simulink model "control_pos_6dof_conMI"  (R2023b)
settings: Solver=ode45  StartTime=0.0  StopTime=tsim  FixedStep=tstep  MaxStep=tstep
undefined symbols (not defined in the file): a0, a1, MI_Contr1, MI_Contr2, MI_Contr3, MI_Contr4, MI_Contr5, MI_Contr6, MI_motor1, MI_motor2, MI_motor3, MI_motor4, MI_motor5, MI_motor6, robot_params, sigbuilder_block, t_qeq_init, t_tr_init, tau_L, tr_ref
(part 1 of 10)
settings Model: Creator=HP  LastModifiedBy=HP

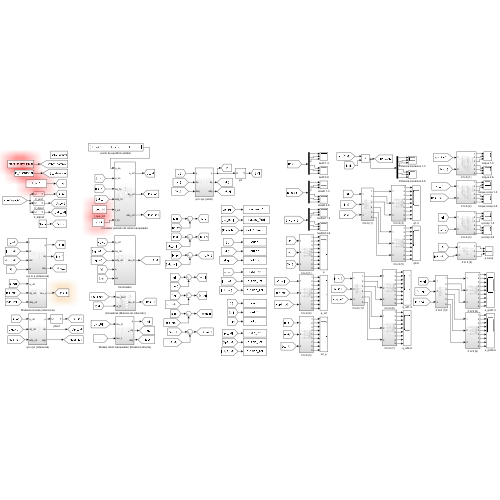
[thumbnail: Simulink's stored preview of the top-level diagram]
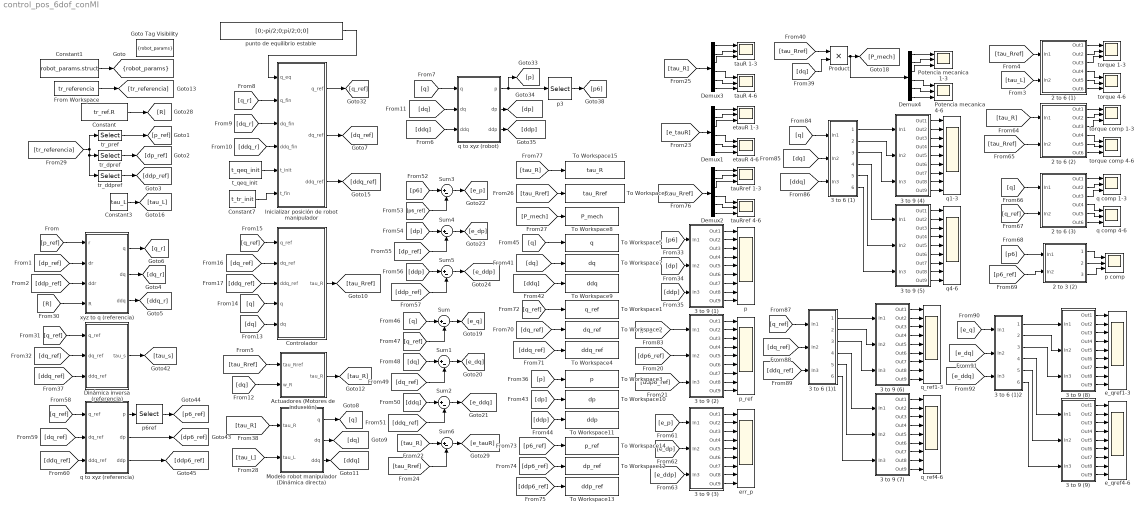
== system control_pos_6dof_conMI ==
  2 to 3 (2) : Subsystem
  2 to 6 (1) : Subsystem
  2 to 6 (2) : Subsystem
  2 to 6 (3) : Subsystem
  3 to 6 (1) : Subsystem
  3 to 6 (1)1 : Subsystem
  3 to 6 (1)2 : Subsystem
  3 to 9 (1) : Subsystem
  3 to 9 (2) : Subsystem
  3 to 9 (3) : Subsystem
  3 to 9 (4) : Subsystem
  3 to 9 (5) : Subsystem
  3 to 9 (6) : Subsystem
  3 to 9 (7) : Subsystem
  3 to 9 (8) : Subsystem
  3 to 9 (9) : Subsystem
  Actuadores (Motores de inducción) : Subsystem
  Constant : Constant  Value=tr_ref.R
  Constant1 : Constant  Value=robot_params.struct  OutDataTypeStr=Bus: robot_params_bus
  Constant3 : Constant  Value=tau_L
  Constant7 : Constant  Value=t_tr_init
  Controlador : Subsystem
  Demux{1..4} (4 alike) : Demux  Outputs=6
  Dinámica inversa (referencia) : Subsystem
  From Workspace : FromWorkspace  VariableName=tr_referencia
  Goto Tag Visibility : GotoTagVisibility  GotoTag=robot_params
  Inicializar posición de robot manipulador : Subsystem
  Modelo robot manipulador (Dinámica directa) : Subsystem
  Potencia mecanica 1-3 : Scope  NumInputPorts=3
  Potencia mecanica 4-6 : Scope  NumInputPorts=3
  Product : Product
  Sum{,1..6} (7 alike) : Sum  Inputs=|+-
  To Workspace1 : ToWorkspace  VariableName=q_ref  SaveFormat=Timeseries  SampleTime=-1
  To Workspace10 : ToWorkspace  VariableName=dp  SaveFormat=Timeseries  SampleTime=-1
  To Workspace11 : ToWorkspace  VariableName=ddp  SaveFormat=Timeseries  SampleTime=-1
  To Workspace12 : ToWorkspace  VariableName=dp_ref  SaveFormat=Timeseries  SampleTime=-1
  To Workspace13 : ToWorkspace  VariableName=ddp_ref  SaveFormat=Timeseries  SampleTime=-1
  To Workspace14 : ToWorkspace  VariableName=p_ref  SaveFormat=Timeseries  SampleTime=-1
  To Workspace15 : ToWorkspace  VariableName=tau_R  SaveFormat=Timeseries  SampleTime=-1
  To Workspace2 : ToWorkspace  VariableName=dq_ref  SaveFormat=Timeseries  SampleTime=-1
  To Workspace3 : ToWorkspace  VariableName=p  SaveFormat=Timeseries  SampleTime=-1
  To Workspace4 : ToWorkspace  VariableName=ddq_ref  SaveFormat=Timeseries  SampleTime=-1
  To Workspace5 : ToWorkspace  VariableName=q  SaveFormat=Timeseries  SampleTime=-1
  To Workspace6 : ToWorkspace  VariableName=tau_Rref  SaveFormat=Timeseries  SampleTime=-1
  To Workspace7 : ToWorkspace  VariableName=dq  SaveFormat=Timeseries  SampleTime=-1
  To Workspace8 : ToWorkspace  VariableName=P_mech  SaveFormat=Timeseries  SampleTime=-1
  To Workspace9 : ToWorkspace  VariableName=ddq  SaveFormat=Timeseries  SampleTime=-1
  e_qref1-3 : Scope  NumInputPorts=9
  e_qref4-6 : Scope  NumInputPorts=9
  err_p : Scope  NumInputPorts=9
  etauR 1-3 : Scope  NumInputPorts=3
  etauR 4-6 : Scope  NumInputPorts=3
  p : Scope  NumInputPorts=9
  p comp : Scope  NumInputPorts=3
  p3 : Selector  NumberOfDimensions=2  InputPortWidth=3  IndexOptions=Index vector (dialog),Index vector (dialog)  Indices=[1:3],6  OutputSizes=1,1
  p6ref : Selector  NumberOfDimensions=2  InputPortWidth=3  IndexOptions=Index vector (dialog),Index vector (dialog)  Indices=[1:3],6  OutputSizes=1,1
  p_ref : Scope  NumInputPorts=9
  punto de equilibrio estable : Constant  Value=[0;-pi/2;0;pi/2;0;0]
  q comp 1-3 : Scope  NumInputPorts=3
  q comp 4-6 : Scope  NumInputPorts=3
  q to xyz (referencia) : Subsystem
  q to xyz (robot) : Subsystem
  q1-3 : Scope  NumInputPorts=9
  q4-6 : Scope  NumInputPorts=9
  q_ref1-3 : Scope  NumInputPorts=9
  q_ref4-6 : Scope  NumInputPorts=9
  t_qeq_init : Constant  Value=t_qeq_init
  tauR 1-3 : Scope  NumInputPorts=3
  tauR 4-6 : Scope  NumInputPorts=3
  tauRref 1-3 : Scope  NumInputPorts=3
  tauRref 4-6 : Scope  NumInputPorts=3
  torque 1-3 : Scope  NumInputPorts=3
  torque 4-6 : Scope  NumInputPorts=3
  torque comp 1-3 : Scope  NumInputPorts=3
  torque comp 4-6 : Scope  NumInputPorts=3
  tr_ddpref : Selector  NumberOfDimensions=2  InputPortWidth=3  IndexOptions=Index vector (dialog),Index vector (dialog)  Indices=[7:9],1  OutputSizes=1,1
  tr_dpref : Selector  NumberOfDimensions=2  InputPortWidth=3  IndexOptions=Index vector (dialog),Index vector (dialog)  Indices=[4:6],1  OutputSizes=1,1
  tr_pref : Selector  NumberOfDimensions=2  InputPortWidth=3  IndexOptions=Index vector (dialog),Index vector (dialog)  Indices=[1:3],1  OutputSizes=1,1
  xyz to q (referencia) : Subsystem
  tag scope: robot_params=scoped
  wires:
  [tr_referencia] -> tr_dpref/1, tr_ddpref/1, tr_pref/1
  3 to 9 (1)/8(Out8) -> p/8
  [ddp] -> 3 to 9 (1)/3(In3)
  [dp] -> 3 to 9 (1)/2(In2)
  3 to 9 (1)/2(Out2) -> p/2
  [p6] -> 3 to 9 (1)/1(In1)
  3 to 9 (1)/7(Out7) -> p/7
  3 to 9 (1)/3(Out3) -> p/3
  3 to 9 (1)/5(Out5) -> p/5
  3 to 9 (1)/6(Out6) -> p/6
  3 to 9 (1)/9(Out9) -> p/9
  3 to 9 (1)/1(Out1) -> p/1
  3 to 9 (1)/4(Out4) -> p/4
  Constant3/1 -> [tau_L]
  [tau_Rref] -> Product/1
  [dq] -> Product/2
  [ddp] -> To Workspace11/1
  [P_mech] -> To Workspace8/1
  [dq] -> To Workspace7/1
  [q] -> To Workspace5/1
  [tau_Rref] -> To Workspace6/1
  [dp] -> To Workspace10/1
  [p] -> To Workspace3/1
  [ddq] -> To Workspace9/1
  [q] -> Sum/1
  [q_ref] -> Sum/2
  Sum/1 -> [e_q]
  [dq_ref] -> Sum1/2
  Sum1/1 -> [e_dq]
  [dq] -> Sum1/1
  [ddq_ref] -> Sum2/2
  Sum2/1 -> [e_ddq]
  [ddq] -> Sum2/1
  [p6_ref] -> Sum3/2
  Sum4/1 -> [e_dp]
  Sum5/1 -> [e_ddp]
  [ddp_ref] -> Sum5/2
  [dp_ref] -> Sum4/2
  Sum3/1 -> [e_p]
  [p6] -> Sum3/1
  [ddp] -> Sum5/1
  [dp] -> Sum4/1
  3 to 9 (3)/4(Out4) -> err_p/4
  3 to 9 (3)/1(Out1) -> err_p/1
  3 to 9 (3)/3(Out3) -> err_p/3
  3 to 9 (3)/7(Out7) -> err_p/7
  3 to 9 (3)/2(Out2) -> err_p/2
  3 to 9 (3)/6(Out6) -> err_p/6
  3 to 9 (3)/5(Out5) -> err_p/5
  [e_p] -> 3 to 9 (3)/1(In1)
  [e_dp] -> 3 to 9 (3)/2(In2)
  3 to 9 (3)/8(Out8) -> err_p/8
  3 to 9 (3)/9(Out9) -> err_p/9
  [e_ddp] -> 3 to 9 (3)/3(In3)
  [tau_R] -> 2 to 6 (2)/1(In1)
  [tau_Rref] -> 2 to 6 (2)/2(In2)
  [q_ref] -> 2 to 6 (3)/2(In2)
  [q] -> 2 to 6 (3)/1(In1)
  [p6] -> 2 to 3 (2)/1(In1)
  [p6_ref] -> 2 to 3 (2)/2(In2)
  [dq_ref] -> To Workspace2/1
  [ddq_ref] -> To Workspace4/1
  [q_ref] -> To Workspace1/1
  [p6_ref] -> To Workspace14/1
  [dp6_ref] -> To Workspace12/1
  [ddp6_ref] -> To Workspace13/1
  3 to 9 (2)/4(Out4) -> p_ref/4
  3 to 9 (2)/1(Out1) -> p_ref/1
  3 to 9 (2)/3(Out3) -> p_ref/3
  3 to 9 (2)/7(Out7) -> p_ref/7
  3 to 9 (2)/2(Out2) -> p_ref/2
  3 to 9 (2)/6(Out6) -> p_ref/6
  3 to 9 (2)/5(Out5) -> p_ref/5
  [p6_ref] -> 3 to 9 (2)/1(In1)
  3 to 9 (2)/8(Out8) -> p_ref/8
  3 to 9 (2)/9(Out9) -> p_ref/9
  2 to 6 (1)/3(Out3) -> torque 1-3/3
  2 to 6 (1)/2(Out2) -> torque 1-3/2
  2 to 6 (1)/1(Out1) -> torque 1-3/1
  [tau_R] -> Modelo robot manipulador (Dinámica directa)/1(tau_R)
  2 to 6 (1)/6(Out6) -> torque 4-6/3
  [tau_L] -> Modelo robot manipulador (Dinámica directa)/2(tau_L)
  2 to 6 (1)/5(Out5) -> torque 4-6/2
  2 to 6 (1)/4(Out4) -> torque 4-6/1
  Demux2/5 -> tauRref 4-6/2
  Demux2/4 -> tauRref 4-6/1
  [tau_Rref] -> Demux2/1
  Demux2/1 -> tauRref 1-3/1
  Demux2/2 -> tauRref 1-3/2
  Demux2/3 -> tauRref 1-3/3
  Demux2/6 -> tauRref 4-6/3
  3 to 9 (4)/5(Out5) -> q1-3/5
  3 to 9 (4)/2(Out2) -> q1-3/2
  3 to 6 (1)/1(Out1) -> 3 to 9 (4)/1(In1)
  3 to 9 (5)/5(Out5) -> q4-6/5
  3 to 9 (4)/3(Out3) -> q1-3/3
  3 to 9 (5)/3(Out3) -> q4-6/3
  3 to 9 (4)/4(Out4) -> q1-3/4
  3 to 9 (4)/8(Out8) -> q1-3/8
  3 to 9 (4)/7(Out7) -> q1-3/7
  3 to 9 (4)/6(Out6) -> q1-3/6
  3 to 9 (4)/9(Out9) -> q1-3/9
  3 to 9 (5)/1(Out1) -> q4-6/1
  3 to 9 (5)/6(Out6) -> q4-6/6
  3 to 9 (5)/7(Out7) -> q4-6/7
  3 to 9 (5)/4(Out4) -> q4-6/4
  3 to 9 (4)/1(Out1) -> q1-3/1
  3 to 9 (5)/8(Out8) -> q4-6/8
  [q] -> 3 to 6 (1)/1(In1)
  [dq] -> 3 to 6 (1)/2(In2)
  3 to 6 (1)/2(Out2) -> 3 to 9 (4)/2(In2)
  [ddq] -> 3 to 6 (1)/3(In3)
  3 to 6 (1)/3(Out3) -> 3 to 9 (4)/3(In3)
  3 to 9 (5)/2(Out2) -> q4-6/2
  3 to 6 (1)/6(Out6) -> 3 to 9 (5)/3(In3)
  3 to 6 (1)/5(Out5) -> 3 to 9 (5)/2(In2)
  3 to 6 (1)/4(Out4) -> 3 to 9 (5)/1(In1)
  [ddq_ref] -> 3 to 6 (1)1/3(In3)
  3 to 6 (1)1/3(Out3) -> 3 to 9 (6)/3(In3)
  [dq_ref] -> 3 to 6 (1)1/2(In2)
  [q_ref] -> 3 to 6 (1)1/1(In1)
  3 to 9 (7)/8(Out8) -> q_ref4-6/8
  3 to 9 (6)/1(Out1) -> q_ref1-3/1
  3 to 9 (7)/4(Out4) -> q_ref4-6/4
  3 to 6 (1)1/2(Out2) -> 3 to 9 (6)/2(In2)
  3 to 6 (1)1/5(Out5) -> 3 to 9 (7)/2(In2)
  3 to 9 (7)/2(Out2) -> q_ref4-6/2
  3 to 6 (1)1/6(Out6) -> 3 to 9 (7)/3(In3)
  3 to 9 (7)/7(Out7) -> q_ref4-6/7
  3 to 9 (7)/6(Out6) -> q_ref4-6/6
  3 to 9 (7)/1(Out1) -> q_ref4-6/1
  3 to 9 (6)/8(Out8) -> q_ref1-3/8
  3 to 9 (6)/6(Out6) -> q_ref1-3/6
  3 to 9 (6)/7(Out7) -> q_ref1-3/7
  3 to 9 (7)/5(Out5) -> q_ref4-6/5
  3 to 9 (6)/3(Out3) -> q_ref1-3/3
  3 to 9 (7)/3(Out3) -> q_ref4-6/3
  3 to 6 (1)1/1(Out1) -> 3 to 9 (6)/1(In1)
  3 to 9 (6)/2(Out2) -> q_ref1-3/2
  3 to 9 (6)/5(Out5) -> q_ref1-3/5
  3 to 9 (6)/9(Out9) -> q_ref1-3/9
  3 to 9 (6)/4(Out4) -> q_ref1-3/4
  3 to 6 (1)1/4(Out4) -> 3 to 9 (7)/1(In1)
  [e_ddq] -> 3 to 6 (1)2/3(In3)
  3 to 6 (1)2/3(Out3) -> 3 to 9 (8)/3(In3)
  [e_dq] -> 3 to 6 (1)2/2(In2)
  [e_q] -> 3 to 6 (1)2/1(In1)
  3 to 9 (9)/8(Out8) -> e_qref4-6/8
  3 to 9 (8)/1(Out1) -> e_qref1-3/1
  3 to 9 (9)/4(Out4) -> e_qref4-6/4
  3 to 6 (1)2/2(Out2) -> 3 to 9 (8)/2(In2)
  3 to 6 (1)2/5(Out5) -> 3 to 9 (9)/2(In2)
  3 to 9 (9)/2(Out2) -> e_qref4-6/2
  3 to 6 (1)2/6(Out6) -> 3 to 9 (9)/3(In3)
  3 to 9 (9)/7(Out7) -> e_qref4-6/7
  3 to 9 (9)/6(Out6) -> e_qref4-6/6
  3 to 9 (9)/1(Out1) -> e_qref4-6/1
  3 to 9 (8)/8(Out8) -> e_qref1-3/8
  3 to 9 (8)/6(Out6) -> e_qref1-3/6
  3 to 9 (8)/7(Out7) -> e_qref1-3/7
  3 to 9 (9)/5(Out5) -> e_qref4-6/5
  3 to 9 (8)/3(Out3) -> e_qref1-3/3
  3 to 9 (9)/3(Out3) -> e_qref4-6/3
  3 to 6 (1)2/1(Out1) -> 3 to 9 (8)/1(In1)
  3 to 9 (8)/2(Out2) -> e_qref1-3/2
  3 to 9 (8)/5(Out5) -> e_qref1-3/5
  3 to 9 (8)/9(Out9) -> e_qref1-3/9
  3 to 9 (8)/4(Out4) -> e_qref1-3/4
  3 to 6 (1)2/4(Out4) -> 3 to 9 (9)/1(In1)
  3 to 9 (5)/9(Out9) -> q4-6/9
  3 to 9 (7)/9(Out9) -> q_ref4-6/9
  3 to 9 (9)/9(Out9) -> e_qref4-6/9
  2 to 6 (2)/1(Out1) -> torque comp 1-3/1
  2 to 6 (2)/6(Out6) -> torque comp 4-6/3
  2 to 6 (2)/4(Out4) -> torque comp 4-6/1
  2 to 6 (2)/2(Out2) -> torque comp 1-3/2
  2 to 6 (2)/5(Out5) -> torque comp 4-6/2
  2 to 6 (2)/3(Out3) -> torque comp 1-3/3
  2 to 6 (3)/4(Out4) -> q comp 4-6/1
  2 to 6 (3)/2(Out2) -> q comp 1-3/2
  2 to 6 (3)/5(Out5) -> q comp 4-6/2
  2 to 6 (3)/3(Out3) -> q comp 1-3/3
  2 to 6 (3)/6(Out6) -> q comp 4-6/3
  2 to 6 (3)/1(Out1) -> q comp 1-3/1
  2 to 3 (2)/2(2) -> p comp/2
  2 to 3 (2)/1(1) -> p comp/1
  2 to 3 (2)/3(3) -> p comp/3
  Constant/1 -> [R]
  tr_pref/1 -> [p_ref]
  tr_ddpref/1 -> [ddp_ref]
  tr_dpref/1 -> [dp_ref]
  Constant1/1 -> [robot_params]
  [p_ref] -> xyz to q (referencia)/1(r)
  [dp_ref] -> xyz to q (referencia)/2(dr)
  [ddp_ref] -> xyz to q (referencia)/3(ddr)
  [R] -> xyz to q (referencia)/4(R)
  From Workspace/1 -> [tr_referencia]
  p3/1 -> [p6]
  q to xyz (robot)/1(p) -> p3/1, [p]
  [q] -> q to xyz (robot)/1(q)
  [dq] -> q to xyz (robot)/2(dq)
  [ddq] -> q to xyz (robot)/3(ddq)
  q to xyz (robot)/2(dp) -> [dp]
  q to xyz (robot)/3(ddp) -> [ddp]
  Modelo robot manipulador (Dinámica directa)/3(ddq) -> [ddq]
  Modelo robot manipulador (Dinámica directa)/2(dq) -> [dq]
  Modelo robot manipulador (Dinámica directa)/1(q) -> [q]
  [q_ref] -> Controlador/1(q_ref)
  [dq_ref] -> Controlador/2(dq_ref)
  [ddq_ref] -> Controlador/3(ddq_ref)
  [q] -> Controlador/4(q)
  [dq] -> Controlador/5(dq)
  Controlador/1(tau_R) -> [tau_Rref]
  [tau_Rref] -> 2 to 6 (1)/1(In1)
  [tau_L] -> 2 to 6 (1)/2(In2)
  xyz to q (referencia)/2(dq) -> [dq_r]
  xyz to q (referencia)/1(q) -> [q_r]
  xyz to q (referencia)/3(ddq) -> [ddq_r]
  [tau_Rref] -> Sum6/2
  [tau_R] -> Sum6/1
  Sum6/1 -> [e_tauR]
  [dp6_ref] -> 3 to 9 (2)/2(In2)
  [ddp6_ref] -> 3 to 9 (2)/3(In3)
  Demux1/1 -> etauR 1-3/1
  Demux1/3 -> etauR 1-3/3
  Demux1/6 -> etauR 4-6/3
  Demux1/2 -> etauR 1-3/2
  [e_tauR] -> Demux1/1
  Demux1/5 -> etauR 4-6/2
  Demux1/4 -> etauR 4-6/1
  Demux3/3 -> tauR 1-3/3
  Demux3/1 -> tauR 1-3/1
  Demux3/5 -> tauR 4-6/2
  Demux3/2 -> tauR 1-3/2
  Demux3/4 -> tauR 4-6/1
  Demux3/6 -> tauR 4-6/3
  [tau_R] -> Demux3/1
  Dinámica inversa (referencia)/1(tau_s) -> [tau_s]
  q to xyz (referencia)/2(dp) -> [dp6_ref]
  q to xyz (referencia)/3(ddp) -> [ddp6_ref]
  q to xyz (referencia)/1(p) -> p6ref/1
  p6ref/1 -> [p6_ref]
  [q_ref] -> Dinámica inversa (referencia)/1(q_ref)
  [dq_ref] -> Dinámica inversa (referencia)/2(dq_ref)
  [ddq_ref] -> Dinámica inversa (referencia)/3(ddq_ref)
  [q_ref] -> q to xyz (referencia)/1(q_ref)
  [dq_ref] -> q to xyz (referencia)/2(dq_ref)
  [ddq_ref] -> q to xyz (referencia)/3(ddq_ref)
  [tau_R] -> To Workspace15/1
  Demux4/6 -> Potencia mecanica 4-6/3
  Demux4/4 -> Potencia mecanica 4-6/1
  Product/1 -> Demux4/1, [P_mech]
  Demux4/3 -> Potencia mecanica 1-3/3
  Demux4/2 -> Potencia mecanica 1-3/2
  Demux4/1 -> Potencia mecanica 1-3/1
  Demux4/5 -> Potencia mecanica 4-6/2
  Constant7/1 -> Inicializar posición de robot manipulador/6(t_fin)
  [q_r] -> Inicializar posición de robot manipulador/2(q_fin)
  punto de equilibrio estable/1 -> Inicializar posición de robot manipulador/1(q_eq)
  Inicializar posición de robot manipulador/2(dq_ref) -> [dq_ref]
  t_qeq_init/1 -> Inicializar posición de robot manipulador/5(t_init)
  [ddq_r] -> Inicializar posición de robot manipulador/4(ddq_fin)
  Inicializar posición de robot manipulador/1(q_ref) -> [q_ref]
  Inicializar posición de robot manipulador/3(ddq_ref) -> [ddq_ref]
  [dq_r] -> Inicializar posición de robot manipulador/3(dq_fin)
  [tau_Rref] -> Actuadores (Motores de inducción)/1(tau_Rref)
  [dq] -> Actuadores (Motores de inducción)/2(w_R)
  Actuadores (Motores de inducción)/1(tau_R) -> [tau_R]

== system control_pos_6dof_conMI/2 to 3 (2) ==
  In1 : Inport
  In2 : Inport  Port=2
  Demux3 : Demux  Outputs=3
  Demux4 : Demux  Outputs=3
  Mux10 : Mux  Inputs=2
  Mux8 : Mux  Inputs=2
  Mux9 : Mux  Inputs=2
  1 : Outport
  2 : Outport  Port=2
  3 : Outport  Port=3
  wires:
  Demux4/3 -> Mux10/2
  Demux3/1 -> Mux8/1
  Demux3/2 -> Mux9/1
  Mux9/1 -> 2/1
  Demux4/2 -> Mux9/2
  Demux4/1 -> Mux8/2
  Demux3/3 -> Mux10/1
  Mux8/1 -> 1/1
  Mux10/1 -> 3/1
  In1/1 -> Demux3/1
  In2/1 -> Demux4/1

== system control_pos_6dof_conMI/2 to 6 (1) ==
  In1 : Inport
  In2 : Inport  Port=2
  Demux4 : Demux  Outputs=6
  Demux6 : Demux  Outputs=6
  Mux{,1..5} (6 alike) : Mux  Inputs=2
  Out1 : Outport
  Out2 : Outport  Port=2
  Out3 : Outport  Port=3
  Out4 : Outport  Port=4
  Out5 : Outport  Port=5
  Out6 : Outport  Port=6
  wires:
  In2/1 -> Demux6/1
  Demux4/3 -> Mux2/1
  Demux4/5 -> Mux4/1
  Demux4/6 -> Mux5/1
  Demux6/5 -> Mux4/2
  Demux4/1 -> Mux/1
  Demux6/6 -> Mux5/2
  In1/1 -> Demux4/1
  Demux4/4 -> Mux3/1
  Demux6/2 -> Mux1/2
  Demux6/4 -> Mux3/2
  Demux6/1 -> Mux/2
  Demux4/2 -> Mux1/1
  Demux6/3 -> Mux2/2
  Mux/1 -> Out1/1
  Mux1/1 -> Out2/1
  Mux2/1 -> Out3/1
  Mux3/1 -> Out4/1
  Mux4/1 -> Out5/1
  Mux5/1 -> Out6/1

== system control_pos_6dof_conMI/2 to 6 (2) ==
  In1 : Inport
  In2 : Inport  Port=2
  Demux4 : Demux  Outputs=6
  Demux6 : Demux  Outputs=6
  Mux{,1..5} (6 alike) : Mux  Inputs=2
  Out1 : Outport
  Out2 : Outport  Port=2
  Out3 : Outport  Port=3
  Out4 : Outport  Port=4
  Out5 : Outport  Port=5
  Out6 : Outport  Port=6
  wires:
  In2/1 -> Demux6/1
  Demux4/3 -> Mux2/1
  Demux4/5 -> Mux4/1
  Demux4/6 -> Mux5/1
  Demux6/5 -> Mux4/2
  Demux4/1 -> Mux/1
  Demux6/6 -> Mux5/2
  In1/1 -> Demux4/1
  Demux4/4 -> Mux3/1
  Demux6/2 -> Mux1/2
  Demux6/4 -> Mux3/2
  Demux6/1 -> Mux/2
  Demux4/2 -> Mux1/1
  Demux6/3 -> Mux2/2
  Mux/1 -> Out1/1
  Mux1/1 -> Out2/1
  Mux2/1 -> Out3/1
  Mux3/1 -> Out4/1
  Mux4/1 -> Out5/1
  Mux5/1 -> Out6/1

== system control_pos_6dof_conMI/2 to 6 (3) ==
  In1 : Inport
  In2 : Inport  Port=2
  Demux4 : Demux  Outputs=6
  Demux6 : Demux  Outputs=6
  Mux{,1..5} (6 alike) : Mux  Inputs=2
  Out1 : Outport
  Out2 : Outport  Port=2
  Out3 : Outport  Port=3
  Out4 : Outport  Port=4
  Out5 : Outport  Port=5
  Out6 : Outport  Port=6
  wires:
  In2/1 -> Demux6/1
  Demux4/3 -> Mux2/1
  Demux4/5 -> Mux4/1
  Demux4/6 -> Mux5/1
  Demux6/5 -> Mux4/2
  Demux4/1 -> Mux/1
  Demux6/6 -> Mux5/2
  In1/1 -> Demux4/1
  Demux4/4 -> Mux3/1
  Demux6/2 -> Mux1/2
  Demux6/4 -> Mux3/2
  Demux6/1 -> Mux/2
  Demux4/2 -> Mux1/1
  Demux6/3 -> Mux2/2
  Mux/1 -> Out1/1
  Mux1/1 -> Out2/1
  Mux2/1 -> Out3/1
  Mux3/1 -> Out4/1
  Mux4/1 -> Out5/1
  Mux5/1 -> Out6/1

== system control_pos_6dof_conMI/3 to 6 (1) ==
  In1 : Inport
  In2 : Inport  Port=2
  In3 : Inport  Port=3
  Demux4 : Demux  Outputs=6
  Demux6 : Demux  Outputs=6
  Demux7 : Demux  Outputs=6
  Mux{,1..5} (6 alike) : Mux  Inputs=3
  Out1 : Outport
  Out2 : Outport  Port=2
  Out3 : Outport  Port=3
  Out4 : Outport  Port=4
  Out5 : Outport  Port=5
  Out6 : Outport  Port=6
  wires:
  Demux6/1 -> Mux2/1
  Demux6/3 -> Mux2/3
  Demux4/2 -> Mux/2
  Demux6/6 -> Mux3/3
  Demux6/2 -> Mux2/2
  Demux6/5 -> Mux3/2
  Mux/1 -> Out1/1
  In1/1 -> Demux4/1
  Demux6/4 -> Mux3/1
  Demux4/1 -> Mux/1
  Demux4/6 -> Mux1/3
  Demux4/4 -> Mux1/1
  Demux7/5 -> Mux5/2
  Demux4/3 -> Mux/3
  Demux4/5 -> Mux1/2
  Demux7/3 -> Mux4/3
  Demux7/1 -> Mux4/1
  Demux7/2 -> Mux4/2
  In3/1 -> Demux7/1
  Mux2/1 -> Out2/1
  Demux7/4 -> Mux5/1
  Demux7/6 -> Mux5/3
  In2/1 -> Demux6/1
  Mux5/1 -> Out6/1
  Mux1/1 -> Out4/1
  Mux4/1 -> Out3/1
  Mux3/1 -> Out5/1

== system control_pos_6dof_conMI/3 to 6 (1)1 ==
  In1 : Inport
  In2 : Inport  Port=2
  In3 : Inport  Port=3
  Demux4 : Demux  Outputs=6
  Demux6 : Demux  Outputs=6
  Demux7 : Demux  Outputs=6
  Mux{,1..5} (6 alike) : Mux  Inputs=3
  Out1 : Outport
  Out2 : Outport  Port=2
  Out3 : Outport  Port=3
  Out4 : Outport  Port=4
  Out5 : Outport  Port=5
  Out6 : Outport  Port=6
  wires:
  Demux6/1 -> Mux2/1
  Demux6/3 -> Mux2/3
  Demux4/2 -> Mux/2
  Demux6/6 -> Mux3/3
  Demux6/2 -> Mux2/2
  Demux6/5 -> Mux3/2
  Mux/1 -> Out1/1
  In1/1 -> Demux4/1
  Demux6/4 -> Mux3/1
  Demux4/1 -> Mux/1
  Demux4/6 -> Mux1/3
  Demux4/4 -> Mux1/1
  Demux7/5 -> Mux5/2
  Demux4/3 -> Mux/3
  Demux4/5 -> Mux1/2
  Demux7/3 -> Mux4/3
  Demux7/1 -> Mux4/1
  Demux7/2 -> Mux4/2
  In3/1 -> Demux7/1
  Mux2/1 -> Out2/1
  Demux7/4 -> Mux5/1
  Demux7/6 -> Mux5/3
  In2/1 -> Demux6/1
  Mux5/1 -> Out6/1
  Mux1/1 -> Out4/1
  Mux4/1 -> Out3/1
  Mux3/1 -> Out5/1

== system control_pos_6dof_conMI/3 to 6 (1)2 ==
  In1 : Inport
  In2 : Inport  Port=2
  In3 : Inport  Port=3
  Demux4 : Demux  Outputs=6
  Demux6 : Demux  Outputs=6
  Demux7 : Demux  Outputs=6
  Mux{,1..5} (6 alike) : Mux  Inputs=3
  Out1 : Outport
  Out2 : Outport  Port=2
  Out3 : Outport  Port=3
  Out4 : Outport  Port=4
  Out5 : Outport  Port=5
  Out6 : Outport  Port=6
  wires:
  Demux6/1 -> Mux2/1
  Demux6/3 -> Mux2/3
  Demux4/2 -> Mux/2
  Demux6/6 -> Mux3/3
  Demux6/2 -> Mux2/2
  Demux6/5 -> Mux3/2
  Mux/1 -> Out1/1
  In1/1 -> Demux4/1
  Demux6/4 -> Mux3/1
  Demux4/1 -> Mux/1
  Demux4/6 -> Mux1/3
  Demux4/4 -> Mux1/1
  Demux7/5 -> Mux5/2
  Demux4/3 -> Mux/3
  Demux4/5 -> Mux1/2
  Demux7/3 -> Mux4/3
  Demux7/1 -> Mux4/1
  Demux7/2 -> Mux4/2
  In3/1 -> Demux7/1
  Mux2/1 -> Out2/1
  Demux7/4 -> Mux5/1
  Demux7/6 -> Mux5/3
  In2/1 -> Demux6/1
  Mux5/1 -> Out6/1
  Mux1/1 -> Out4/1
  Mux4/1 -> Out3/1
  Mux3/1 -> Out5/1

== system control_pos_6dof_conMI/3 to 9 (1) ==
  In1 : Inport
  In2 : Inport  Port=2
  In3 : Inport  Port=3
  Demux2 : Demux  Outputs=3
  Demux3 : Demux  Outputs=3
  Demux4 : Demux  Outputs=3
  Out1 : Outport
  Out2 : Outport  Port=2
  Out3 : Outport  Port=3
  Out4 : Outport  Port=4
  Out5 : Outport  Port=5
  Out6 : Outport  Port=6
  Out7 : Outport  Port=7
  Out8 : Outport  Port=8
  Out9 : Outport  Port=9
  wires:
  In3/1 -> Demux4/1
  Demux4/1 -> Out3/1
  Demux2/1 -> Out1/1
  Demux3/3 -> Out8/1
  Demux3/2 -> Out5/1
  Demux3/1 -> Out2/1
  In1/1 -> Demux2/1
  Demux2/3 -> Out7/1
  Demux4/3 -> Out9/1
  Demux4/2 -> Out6/1
  Demux2/2 -> Out4/1
  In2/1 -> Demux3/1

== system control_pos_6dof_conMI/3 to 9 (2) ==
  In1 : Inport
  In2 : Inport  Port=2
  In3 : Inport  Port=3
  Demux2 : Demux  Outputs=3
  Demux3 : Demux  Outputs=3
  Demux4 : Demux  Outputs=3
  Out1 : Outport
  Out2 : Outport  Port=2
  Out3 : Outport  Port=3
  Out4 : Outport  Port=4
  Out5 : Outport  Port=5
  Out6 : Outport  Port=6
  Out7 : Outport  Port=7
  Out8 : Outport  Port=8
  Out9 : Outport  Port=9
  wires:
  In3/1 -> Demux4/1
  Demux4/1 -> Out3/1
  Demux2/1 -> Out1/1
  Demux3/3 -> Out8/1
  Demux3/2 -> Out5/1
  Demux3/1 -> Out2/1
  In1/1 -> Demux2/1
  Demux2/3 -> Out7/1
  Demux4/3 -> Out9/1
  Demux4/2 -> Out6/1
  Demux2/2 -> Out4/1
  In2/1 -> Demux3/1

== system control_pos_6dof_conMI/3 to 9 (3) ==
  In1 : Inport
  In2 : Inport  Port=2
  In3 : Inport  Port=3
  Demux2 : Demux  Outputs=3
  Demux3 : Demux  Outputs=3
  Demux4 : Demux  Outputs=3
  Out1 : Outport
  Out2 : Outport  Port=2
  Out3 : Outport  Port=3
  Out4 : Outport  Port=4
  Out5 : Outport  Port=5
  Out6 : Outport  Port=6
  Out7 : Outport  Port=7
  Out8 : Outport  Port=8
  Out9 : Outport  Port=9
  wires:
  In3/1 -> Demux4/1
  Demux4/1 -> Out3/1
  Demux2/1 -> Out1/1
  Demux3/3 -> Out8/1
  Demux3/2 -> Out5/1
  Demux3/1 -> Out2/1
  In1/1 -> Demux2/1
  Demux2/3 -> Out7/1
  Demux4/3 -> Out9/1
  Demux4/2 -> Out6/1
  Demux2/2 -> Out4/1
  In2/1 -> Demux3/1

== system control_pos_6dof_conMI/3 to 9 (4) ==
  In1 : Inport
  In2 : Inport  Port=2
  In3 : Inport  Port=3
  Demux2 : Demux  Outputs=3
  Demux3 : Demux  Outputs=3
  Demux4 : Demux  Outputs=3
  Out1 : Outport
  Out2 : Outport  Port=2
  Out3 : Outport  Port=3
  Out4 : Outport  Port=4
  Out5 : Outport  Port=5
  Out6 : Outport  Port=6
  Out7 : Outport  Port=7
  Out8 : Outport  Port=8
  Out9 : Outport  Port=9
  wires:
  In3/1 -> Demux4/1
  Demux4/1 -> Out3/1
  Demux2/1 -> Out1/1
  Demux3/3 -> Out8/1
  Demux3/2 -> Out5/1
  Demux3/1 -> Out2/1
  In1/1 -> Demux2/1
  Demux2/3 -> Out7/1
  Demux4/3 -> Out9/1
  Demux4/2 -> Out6/1
  Demux2/2 -> Out4/1
  In2/1 -> Demux3/1

== system control_pos_6dof_conMI/3 to 9 (5) ==
  In1 : Inport
  In2 : Inport  Port=2
  In3 : Inport  Port=3
  Demux2 : Demux  Outputs=3
  Demux3 : Demux  Outputs=3
  Demux4 : Demux  Outputs=3
  Out1 : Outport
  Out2 : Outport  Port=2
  Out3 : Outport  Port=3
  Out4 : Outport  Port=4
  Out5 : Outport  Port=5
  Out6 : Outport  Port=6
  Out7 : Outport  Port=7
  Out8 : Outport  Port=8
  Out9 : Outport  Port=9
  wires:
  In3/1 -> Demux4/1
  Demux4/1 -> Out3/1
  Demux2/1 -> Out1/1
  Demux3/3 -> Out8/1
  Demux3/2 -> Out5/1
  Demux3/1 -> Out2/1
  In1/1 -> Demux2/1
  Demux2/3 -> Out7/1
  Demux4/3 -> Out9/1
  Demux4/2 -> Out6/1
  Demux2/2 -> Out4/1
  In2/1 -> Demux3/1

== system control_pos_6dof_conMI/3 to 9 (6) ==
  In1 : Inport
  In2 : Inport  Port=2
  In3 : Inport  Port=3
  Demux2 : Demux  Outputs=3
  Demux3 : Demux  Outputs=3
  Demux4 : Demux  Outputs=3
  Out1 : Outport
  Out2 : Outport  Port=2
  Out3 : Outport  Port=3
  Out4 : Outport  Port=4
  Out5 : Outport  Port=5
  Out6 : Outport  Port=6
  Out7 : Outport  Port=7
  Out8 : Outport  Port=8
  Out9 : Outport  Port=9
  wires:
  In3/1 -> Demux4/1
  Demux4/1 -> Out3/1
  Demux2/1 -> Out1/1
  Demux3/3 -> Out8/1
  Demux3/2 -> Out5/1
  Demux3/1 -> Out2/1
  In1/1 -> Demux2/1
  Demux2/3 -> Out7/1
  Demux4/3 -> Out9/1
  Demux4/2 -> Out6/1
  Demux2/2 -> Out4/1
  In2/1 -> Demux3/1

== system control_pos_6dof_conMI/3 to 9 (7) ==
  In1 : Inport
  In2 : Inport  Port=2
  In3 : Inport  Port=3
  Demux2 : Demux  Outputs=3
  Demux3 : Demux  Outputs=3
  Demux4 : Demux  Outputs=3
  Out1 : Outport
  Out2 : Outport  Port=2
  Out3 : Outport  Port=3
  Out4 : Outport  Port=4
  Out5 : Outport  Port=5
  Out6 : Outport  Port=6
  Out7 : Outport  Port=7
  Out8 : Outport  Port=8
  Out9 : Outport  Port=9
  wires:
  In3/1 -> Demux4/1
  Demux4/1 -> Out3/1
  Demux2/1 -> Out1/1
  Demux3/3 -> Out8/1
  Demux3/2 -> Out5/1
  Demux3/1 -> Out2/1
  In1/1 -> Demux2/1
  Demux2/3 -> Out7/1
  Demux4/3 -> Out9/1
  Demux4/2 -> Out6/1
  Demux2/2 -> Out4/1
  In2/1 -> Demux3/1

== system control_pos_6dof_conMI/3 to 9 (8) ==
  In1 : Inport
  In2 : Inport  Port=2
  In3 : Inport  Port=3
  Demux2 : Demux  Outputs=3
  Demux3 : Demux  Outputs=3
  Demux4 : Demux  Outputs=3
  Out1 : Outport
  Out2 : Outport  Port=2
  Out3 : Outport  Port=3
  Out4 : Outport  Port=4
  Out5 : Outport  Port=5
  Out6 : Outport  Port=6
  Out7 : Outport  Port=7
  Out8 : Outport  Port=8
  Out9 : Outport  Port=9
  wires:
  In3/1 -> Demux4/1
  Demux4/1 -> Out3/1
  Demux2/1 -> Out1/1
  Demux3/3 -> Out8/1
  Demux3/2 -> Out5/1
  Demux3/1 -> Out2/1
  In1/1 -> Demux2/1
  Demux2/3 -> Out7/1
  Demux4/3 -> Out9/1
  Demux4/2 -> Out6/1
  Demux2/2 -> Out4/1
  In2/1 -> Demux3/1

== system control_pos_6dof_conMI/3 to 9 (9) ==
  In1 : Inport
  In2 : Inport  Port=2
  In3 : Inport  Port=3
  Demux2 : Demux  Outputs=3
  Demux3 : Demux  Outputs=3
  Demux4 : Demux  Outputs=3
  Out1 : Outport
  Out2 : Outport  Port=2
  Out3 : Outport  Port=3
  Out4 : Outport  Port=4
  Out5 : Outport  Port=5
  Out6 : Outport  Port=6
  Out7 : Outport  Port=7
  Out8 : Outport  Port=8
  Out9 : Outport  Port=9
  wires:
  In3/1 -> Demux4/1
  Demux4/1 -> Out3/1
  Demux2/1 -> Out1/1
  Demux3/3 -> Out8/1
  Demux3/2 -> Out5/1
  Demux3/1 -> Out2/1
  In1/1 -> Demux2/1
  Demux2/3 -> Out7/1
  Demux4/3 -> Out9/1
  Demux4/2 -> Out6/1
  Demux2/2 -> Out4/1
  In2/1 -> Demux3/1

== system control_pos_6dof_conMI/Actuadores (Motores de inducción) ==
  tau_Rref : Inport
  w_R : Inport  Port=2
  Demux : Demux  Outputs=6
  Demux3 : Demux  Outputs=6
  MI1 + PBC Torque Controller : Subsystem
  MI2 + PBC Torque Controller : Subsystem
  MI3 + PBC Torque Controller : Subsystem
  MI4 + PBC Torque Controller : Subsystem
  MI5 + PBC Torque Controller : Subsystem
  MI6 + PBC Torque Controller : Subsystem
  Mux : Mux  Inputs=6
  tau_R : Outport
  wires:
  Demux3/1 -> MI1 + PBC Torque Controller/2(dq)
  Demux/1 -> MI1 + PBC Torque Controller/1(tau_Rref)
  MI1 + PBC Torque Controller/1(tau_R) -> Mux/1
  Demux3/3 -> MI3 + PBC Torque Controller/2(dq)
  MI2 + PBC Torque Controller/1(tau_R) -> Mux/2
  MI3 + PBC Torque Controller/1(tau_R) -> Mux/3
  Demux3/2 -> MI2 + PBC Torque Controller/2(dq)
  Demux/3 -> MI3 + PBC Torque Controller/1(tau_Rref)
  Demux/2 -> MI2 + PBC Torque Controller/1(tau_Rref)
  tau_Rref/1 -> Demux/1
  w_R/1 -> Demux3/1
  Mux/1 -> tau_R/1
  Demux/4 -> MI4 + PBC Torque Controller/1(tau_Rref)
  Demux/5 -> MI5 + PBC Torque Controller/1(tau_Rref)
  Demux/6 -> MI6 + PBC Torque Controller/1(tau_Rref)
  Demux3/4 -> MI4 + PBC Torque Controller/2(dq)
  Demux3/5 -> MI5 + PBC Torque Controller/2(dq)
  Demux3/6 -> MI6 + PBC Torque Controller/2(dq)
  MI4 + PBC Torque Controller/1(tau_R) -> Mux/4
  MI5 + PBC Torque Controller/1(tau_R) -> Mux/5
  MI6 + PBC Torque Controller/1(tau_R) -> Mux/6

== system control_pos_6dof_conMI/Controlador ==
  q_ref : Inport
  dq_ref : Inport  Port=2
  ddq_ref : Inport  Port=3
  q : Inport  Port=4
  dq : Inport  Port=5
  Constant10 : Constant  Value=a0
  Constant9 : Constant  Value=a1
  Controlador de posición : MATLAB Function  TreatAsAtomicUnit=on
  Controlador no lineal : MATLAB Function  Commented=on  TreatAsAtomicUnit=on
  From12 : From  Commented=on  GotoTag=robot_params  TagVisibility=scoped
  From13 : From  Commented=on  GotoTag=dq_ref
  From14 : From  Commented=on  GotoTag=ddq_ref
  From15 : From  Commented=on  GotoTag=q_ref
  From16 : From  Commented=on  GotoTag=q
  From17 : From  Commented=on  GotoTag=dq
  From18 : From  Commented=on  GotoTag=A1
  From19 : From  Commented=on  GotoTag=A0
  Goto8 : Goto  Commented=on  GotoTag=tau_R
  Modelo dinámico : MATLAB Function  TreatAsAtomicUnit=on
  tau_R : Outport
  wires:
  [dq] -> Modelo dinámico/3(dq)
  [q] -> Modelo dinámico/2(q)
  [robot_params] -> Modelo dinámico/1(robot_params)
  Modelo dinámico/1(robot_din) -> [robot_din]
  q/1 -> [q]
  dq/1 -> [dq]
  [robot_din] -> Controlador de posición/1(robot_din)
  q_ref/1 -> [q_ref]
  dq_ref/1 -> [dq_ref]
  ddq_ref/1 -> [ddq_ref]
  [ddq_ref] -> Controlador de posición/6(ddq_ref)
  [dq_ref] -> Controlador de posición/5(dq_ref)
  [q_ref] -> Controlador de posición/4(q_ref)
  [q] -> Controlador de posición/7(q)
  [dq] -> Controlador de posición/8(dq)
  [a0] -> Controlador de posición/2(A0)
  [a1] -> Controlador de posición/3(A1)
  Controlador de posición/1(tau_R) -> [tau_R]
  [tau_R] -> tau_R/1
  From12/1 -> Controlador no lineal/1(robot_params)
  From16/1 -> Controlador no lineal/5(q)
  From17/1 -> Controlador no lineal/6(dq)
  From13/1 -> Controlador no lineal/3(dq_ref)
  From15/1 -> Controlador no lineal/2(q_ref)
  From14/1 -> Controlador no lineal/4(ddq_ref)
  From19/1 -> Controlador no lineal/7(A0)
  From18/1 -> Controlador no lineal/8(A1)
  Controlador no lineal/1(tau_R) -> Goto8/1
  Constant10/1 -> [a0]
  Constant9/1 -> [a1]

== system control_pos_6dof_conMI/Dinámica inversa (referencia) ==
  q_ref : Inport
  dq_ref : Inport  Port=2
  ddq_ref : Inport  Port=3
  Dinámica inversa : MATLAB Function  TreatAsAtomicUnit=on
  Modelo dinámico : MATLAB Function  TreatAsAtomicUnit=on
  tau_s : Outport
  wires:
  [dq_ref] -> Dinámica inversa/2(dq)
  [ddq_ref] -> Dinámica inversa/3(ddq)
  [robot_din] -> Dinámica inversa/1(robot_din)
  Dinámica inversa/1(tau_s) -> [tau_s]
  [tau_s] -> tau_s/1
  [robot_params] -> Modelo dinámico/1(robot_params)
  [q_ref] -> Modelo dinámico/2(q)
  [dq_ref] -> Modelo dinámico/3(dq)
  Modelo dinámico/1(robot_din) -> [robot_din]
  ddq_ref/1 -> [ddq_ref]
  dq_ref/1 -> [dq_ref]
  q_ref/1 -> [q_ref]

== system control_pos_6dof_conMI/Inicializar posición de robot manipulador ==
  q_eq : Inport
  q_fin : Inport  Port=2
  dq_fin : Inport  Port=3
  ddq_fin : Inport  Port=4
  t_init : Inport  Port=5
  t_fin : Inport  Port=6
  2 to 6 (3) : Subsystem
  Clock : Clock
  Data Store Memory : DataStoreMemory  DataStoreName=q_init  WriteAfterWriteMsg=warning  InitialValue=[0;-pi/2;0;pi/2;0;0]  ShowAdditionalParam=off
  Data Store Read : DataStoreRead  DataStoreName=q_init  IndexOptions=Index vector (dialog)  Indices=1  OutputSizes=1
  Data Store Read1 : DataStoreRead  DataStoreName=q_init  IndexOptions=Index vector (dialog)  Indices=1  OutputSizes=1
  Data Store Write : DataStoreWrite  DataStoreName=q_init  IndexOptions=Index vector (dialog)  Indices=1  OutputSizes=1
  Demux{,1..4} (5 alike) : Demux  Outputs=6
  MATLAB Function : MATLAB Function  TreatAsAtomicUnit=on
  Scope{,1..5} (6 alike) : Scope  NumInputPorts=6
  Sum : Sum  Inputs=+++
  Sum1 : Sum  Inputs=+++
  dq_init : Subsystem
  dq_init1 : Subsystem
  q_init : Subsystem
  q_init_tr : Subsystem
  q_ref : Outport
  dq_ref : Outport  Port=2
  ddq_ref : Outport  Port=3
  wires:
  [ddq_ref] -> ddq_ref/1
  q_fin/1 -> q_init/2(q_init)
  [t_init] -> dq_init/2(t_fin)
  dq_fin/1 -> dq_init/1(qfin)
  [t_init] -> dq_init1/2(t_fin)
  [dq_ref] -> dq_ref/1
  q_eq/1 -> q_init/1(q_eq)
  ddq_fin/1 -> dq_init1/1(qfin)
  [q_ref] -> q_ref/1
  Demux/1 -> Scope/1
  Demux/2 -> Scope/2
  Demux/3 -> Scope/3
  Demux/4 -> Scope/4
  Demux/5 -> Scope/5
  Demux/6 -> Scope/6
  Demux1/1 -> Scope1/1
  Demux1/6 -> Scope1/6
  Demux1/3 -> Scope1/3
  Demux1/2 -> Scope1/2
  Demux1/5 -> Scope1/5
  Demux1/4 -> Scope1/4
  Demux2/1 -> Scope2/1
  Demux2/6 -> Scope2/6
  Demux2/3 -> Scope2/3
  Demux2/2 -> Scope2/2
  Demux2/5 -> Scope2/5
  Demux2/4 -> Scope2/4
  Sum/1 -> [dq_ref], Demux1/1
  Sum1/1 -> Demux2/1, [ddq_ref]
  q_init_tr/1(qpol) -> [q_ref], Demux/1
  [t_init] -> q_init_tr/3(t_fin)
  [t_init] -> MATLAB Function/2(t_init)
  Clock/1 -> MATLAB Function/1(t)
  MATLAB Function/1(qi) -> Demux3/1, Data Store Write/1
  Data Store Read/1 -> q_init_tr/1(q_init)
  Data Store Read1/1 -> MATLAB Function/4(q_init)
  2 to 6 (3)/1(Out1) -> Scope3/1
  [q_r] -> 2 to 6 (3)/1(In1)
  2 to 6 (3)/3(Out3) -> Scope3/3
  2 to 6 (3)/5(Out5) -> Scope3/5
  2 to 6 (3)/6(Out6) -> Scope3/6
  [q_ref] -> 2 to 6 (3)/2(In2)
  2 to 6 (3)/2(Out2) -> Scope3/2
  q_init/1(q_fin) -> [q_r]
  [q_r] -> MATLAB Function/3(q)
  [q_r] -> q_init_tr/2(q_fin)
  t_init/1 -> q_init/3(t_init)
  2 to 6 (3)/4(Out4) -> Scope3/4
  Demux3/4 -> Scope4/4
  Demux3/3 -> Scope4/3
  Demux3/5 -> Scope4/5
  Demux3/1 -> Scope4/1
  Demux3/2 -> Scope4/2
  Demux3/6 -> Scope4/6
  Demux4/3 -> Scope5/3
  Demux4/5 -> Scope5/5
  Demux4/4 -> Scope5/4
  Demux4/2 -> Scope5/2
  Demux4/6 -> Scope5/6
  Demux4/1 -> Scope5/1
  [q_r] -> Demux4/1
  t_fin/1 -> [t_init]
  [t_init] -> q_init/4(t_fin)
  q_init/2(dq_fin) -> Sum/2
  q_init_tr/2(vpol) -> Sum/1
  dq_init/1(qpol) -> Sum/3
  q_init_tr/3(apol) -> Sum1/1
  q_init/3(ddq_fin) -> Sum1/2
  dq_init1/1(qpol) -> Sum1/3

== system control_pos_6dof_conMI/Modelo robot manipulador (Dinámica directa) ==
  tau_R : Inport
  tau_L : Inport  Port=2
  Dinámica directa : MATLAB Function  TreatAsAtomicUnit=on
  Dinámica directa(1) : MATLAB Function  Commented=on  TreatAsAtomicUnit=on
  Modelo dinámico : MATLAB Function  TreatAsAtomicUnit=on
  Scope : Scope
  int_ddq : Integrator  InitialCondition=[0;0;0;0;0;0]
  int_dq : Integrator  InitialCondition=[0;-1.5708;0;1.5708;0;0]
  q : Outport
  dq : Outport  Port=2
  ddq : Outport  Port=3
  wires:
  tau_R/1 -> [tau_R]
  tau_L/1 -> [tau_L]
  [dq] -> Modelo dinámico/3(dq)
  Modelo dinámico/1(robot_din) -> [robot_din]
  [robot_params] -> Modelo dinámico/1(robot_params)
  [q] -> Modelo dinámico/2(q)
  [robot_din] -> Dinámica directa/1(robot_din)
  [dq] -> Dinámica directa/2(dq)
  [tau_R] -> Dinámica directa/3(tau_R)
  [tau_L] -> Dinámica directa/4(tau_L)
  [q] -> q/1
  [dq] -> dq/1
  [ddq] -> ddq/1
  Dinámica directa/1(ddq) -> Scope/1, [ddq], int_ddq/1
  int_dq/1 -> [q]
  int_ddq/1 -> [dq], int_dq/1

== system control_pos_6dof_conMI/q to xyz (referencia) ==
  q_ref : Inport
  dq_ref : Inport  Port=2
  ddq_ref : Inport  Port=3
  Cinemática directa : MATLAB Function  TreatAsAtomicUnit=on
  Jacobiano : MATLAB Function  TreatAsAtomicUnit=on
  ddq to ddp : MATLAB Function  TreatAsAtomicUnit=on
  derivada Jacobiano : MATLAB Function  TreatAsAtomicUnit=on
  dq to dp : MATLAB Function  TreatAsAtomicUnit=on
  p : Outport
  dp : Outport  Port=2
  ddp : Outport  Port=3
  wires:
  [robot_params] -> Cinemática directa/1(robot_params)
  [q_ref] -> Cinemática directa/2(q)
  Cinemática directa/1(p) -> [p_ref]
  [p_ref] -> p/1
  [JPref] -> dq to dp/1(JP)
  [dq_ref] -> dq to dp/2(dq)
  [dJPref] -> ddq to ddp/1(dJP)
  [ddq_ref] -> ddq to ddp/2(ddq)
  dq to dp/1(dp) -> [dp_ref]
  ddq to ddp/1(ddp) -> [ddp_ref]
  [dp_ref] -> dp/1
  [ddp_ref] -> ddp/1
  [dq_ref] -> derivada Jacobiano/3(dq)
  Jacobiano/1(JP) -> [JPref]
  [q_ref] -> Jacobiano/2(q)
  derivada Jacobiano/1(dJP) -> [dJPref]
  [robot_params] -> derivada Jacobiano/1(robot_params)
  [robot_params] -> Jacobiano/1(robot_params)
  [q_ref] -> derivada Jacobiano/2(q)
  q_ref/1 -> [q_ref]
  dq_ref/1 -> [dq_ref]
  ddq_ref/1 -> [ddq_ref]

== system control_pos_6dof_conMI/q to xyz (robot) ==
  q : Inport
  dq : Inport  Port=2
  ddq : Inport  Port=3
  Cinemática directa : MATLAB Function  TreatAsAtomicUnit=on
  Jacobiano : MATLAB Function  TreatAsAtomicUnit=on
  ddq to ddp : MATLAB Function  TreatAsAtomicUnit=on
  derivada Jacobiano : MATLAB Function  TreatAsAtomicUnit=on
  dq to dp : MATLAB Function  TreatAsAtomicUnit=on
  q to xyz : MATLAB Function  Commented=on  TreatAsAtomicUnit=on
  p : Outport
  dp : Outport  Port=2
  ddp : Outport  Port=3
  wires:
  Jacobiano/1(JP) -> [JP]
  [robot_params] -> Jacobiano/1(robot_params)
  [dJP] -> ddq to ddp/1(dJP)
  [robot_params] -> Cinemática directa/1(robot_params)
  [JP] -> dq to dp/1(JP)
  [robot_params] -> derivada Jacobiano/1(robot_params)
  [q] -> Cinemática directa/2(q)
  [dq] -> dq to dp/2(dq)
  derivada Jacobiano/1(dJP) -> [dJP]
  [q] -> derivada Jacobiano/2(q)
  Cinemática directa/1(p) -> p/1
  ddq to ddp/1(ddp) -> ddp/1
  dq to dp/1(dp) -> dp/1
  q/1 -> [q]
  dq/1 -> [dq]
  ddq/1 -> [ddq]
  [q] -> Jacobiano/2(q)
  [dq] -> derivada Jacobiano/3(dq)
  [ddq] -> ddq to ddp/2(ddq)

== system control_pos_6dof_conMI/xyz to q (referencia) ==
  r : Inport
  dr : Inport  Port=2
  ddr : Inport  Port=3
  R : Inport  Port=4
  Cinemática inversa : MATLAB Function  TreatAsAtomicUnit=on
  Jacobiano : MATLAB Function  TreatAsAtomicUnit=on
  ddr to ddq : MATLAB Function  TreatAsAtomicUnit=on
  derivada Jacobiano : MATLAB Function  TreatAsAtomicUnit=on
  dr to dq : MATLAB Function  TreatAsAtomicUnit=on
  q : Outport
  dq : Outport  Port=2
  ddq : Outport  Port=3
  wires:
  R/1 -> [R]
  dr/1 -> [dr]
  ddr/1 -> [ddr]
  r/1 -> [r]
  [robot_params] -> Cinemática inversa/1(robot_params)
  [r] -> Cinemática inversa/2(r)
  [R] -> Cinemática inversa/3(R)
  Cinemática inversa/1(q) -> [q_ref]
  [dq_ref] -> dq/1
  [ddq_ref] -> ddq/1
  [q_ref] -> q/1
  [dr] -> dr to dq/2(dr)
  dr to dq/1(dq) -> [dq_ref]
  [q_ref] -> Jacobiano/2(q)
  Jacobiano/1(JP) -> [JPref]
  [robot_params] -> Jacobiano/1(robot_params)
  [robot_params] -> derivada Jacobiano/1(robot_params)
  derivada Jacobiano/1(dJP) -> [dJPref]
  [q_ref] -> derivada Jacobiano/2(q)
  [dq_ref] -> derivada Jacobiano/3(dq)
  [JPref] -> dr to dq/1(JP)
  [dJPref] -> ddr to ddq/2(dJP)
  ddr to ddq/1(ddq) -> [ddq_ref]
  [ddr] -> ddr to ddq/4(ddr)
  [dq_ref] -> ddr to ddq/3(dq)
  [JPref] -> ddr to ddq/1(JP)

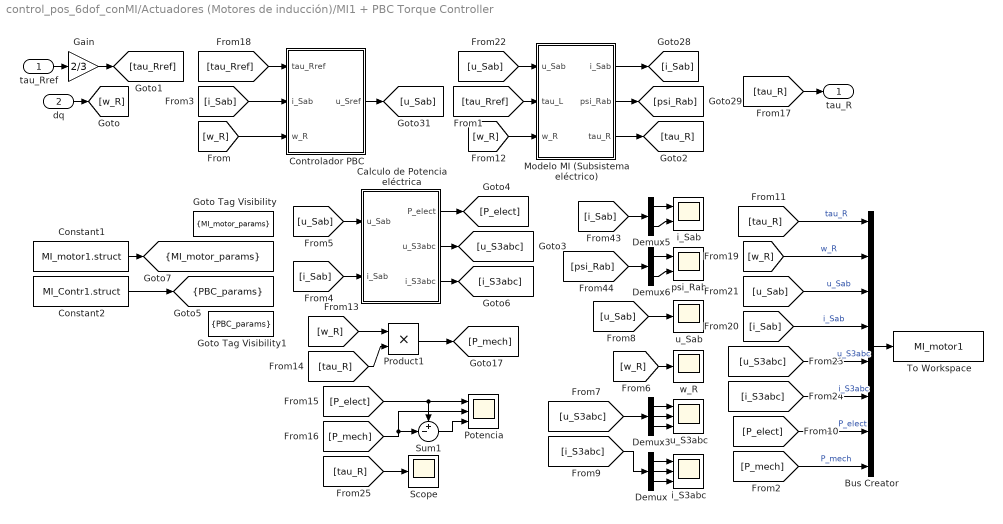
== system control_pos_6dof_conMI/Actuadores (Motores de inducción)/MI1 + PBC Torque Controller ==
  tau_Rref : Inport
  dq : Inport  Port=2
  Bus Creator : BusCreator  Inputs=8
  Calculo de Potencia eléctrica : Subsystem
  Constant1 : Constant  Value=MI_motor1.struct  OutDataTypeStr=Bus: MI_bus
  Constant2 : Constant  Value=MI_Contr1.struct  OutDataTypeStr=Bus: PBC_bus
  Controlador PBC : Subsystem
  Demux : Demux  Outputs=3
  Demux3 : Demux  Outputs=3
  Demux5 : Demux  Outputs=2
  Demux6 : Demux  Outputs=2
  Gain : Gain  Gain=2/3
  Goto Tag Visibility : GotoTagVisibility  GotoTag=MI_motor_params
  Goto Tag Visibility1 : GotoTagVisibility  GotoTag=PBC_params
  Modelo MI (Subsistema eléctrico) : Subsystem
  Potencia : Scope  NumInputPorts=3
  Product1 : Product
  Scope : Scope
  Sum1 : Sum  Inputs=+-|
  To Workspace : ToWorkspace  VariableName=MI_motor1  SaveFormat=Timeseries  SampleTime=-1
  i_S3abc : Scope  NumInputPorts=3
  i_Sab : Scope  NumInputPorts=2
  psi_Rab : Scope  NumInputPorts=2
  u_S3abc : Scope  NumInputPorts=3
  u_Sab : Scope
  w_R : Scope
  tau_R : Outport
  tag scope: MI_motor_params=scoped, PBC_params=scoped
  wires:
  Modelo MI (Subsistema eléctrico)/2(psi_Rab) -> [psi_Rab]
  [u_Sab] -> Modelo MI (Subsistema eléctrico)/1(u_Sab)
  [i_Sab] -> Controlador PBC/2(i_Sab)
  Controlador PBC/1(u_Sref) -> [u_Sab]
  [w_R] -> Controlador PBC/3(w_R)
  [tau_Rref] -> Modelo MI (Subsistema eléctrico)/2(tau_L)
  Calculo de Potencia eléctrica/2(u_S3abc) -> [u_S3abc]
  Calculo de Potencia eléctrica/1(P_elect) -> [P_elect]
  Demux5/1 -> i_Sab/1
  [w_R] -> w_R/1
  [u_Sab] -> Calculo de Potencia eléctrica/1(u_Sab)
  [psi_Rab] -> Demux6/1
  [u_Sab] -> u_Sab/1
  Demux6/1 -> psi_Rab/1
  Calculo de Potencia eléctrica/3(i_S3abc) -> [i_S3abc]
  Demux6/2 -> psi_Rab/2
  Demux5/2 -> i_Sab/2
  [i_Sab] -> Calculo de Potencia eléctrica/2(i_Sab)
  [i_Sab] -> Demux5/1
  Demux/2 -> i_S3abc/2
  Demux3/1 -> u_S3abc/1
  Demux3/3 -> u_S3abc/3
  [i_S3abc] -> Demux/1
  Demux/1 -> i_S3abc/1
  Demux/3 -> i_S3abc/3
  [u_S3abc] -> Demux3/1
  Demux3/2 -> u_S3abc/2
  Modelo MI (Subsistema eléctrico)/1(i_Sab) -> [i_Sab]
  Modelo MI (Subsistema eléctrico)/3(tau_R) -> [tau_R]
  Product1/1 -> [P_mech]
  [w_R] -> Product1/1
  [tau_R] -> Product1/2
  [tau_R] -> Bus Creator/1  "tau_R"
  Sum1/1 -> Potencia/3
  [P_elect] -> Potencia/1, Sum1/1
  [P_mech] -> Potencia/2, Sum1/2
  [tau_R] -> tau_R/1
  dq/1 -> [w_R]
  [tau_Rref] -> Controlador PBC/1(tau_Rref)
  [w_R] -> Modelo MI (Subsistema eléctrico)/3(w_R)
  Bus Creator/1 -> To Workspace/1
  Constant1/1 -> [MI_motor_params]
  [tau_R] -> Scope/1
  Constant2/1 -> [PBC_params]
  [w_R] -> Bus Creator/2  "w_R"
  [u_Sab] -> Bus Creator/3  "u_Sab"
  [i_Sab] -> Bus Creator/4  "i_Sab"
  [u_S3abc] -> Bus Creator/5  "u_S3abc"
  [i_S3abc] -> Bus Creator/6  "i_S3abc"
  [P_elect] -> Bus Creator/7  "P_elect"
  [P_mech] -> Bus Creator/8  "P_mech"
  tau_Rref/1 -> Gain/1
  Gain/1 -> [tau_Rref]

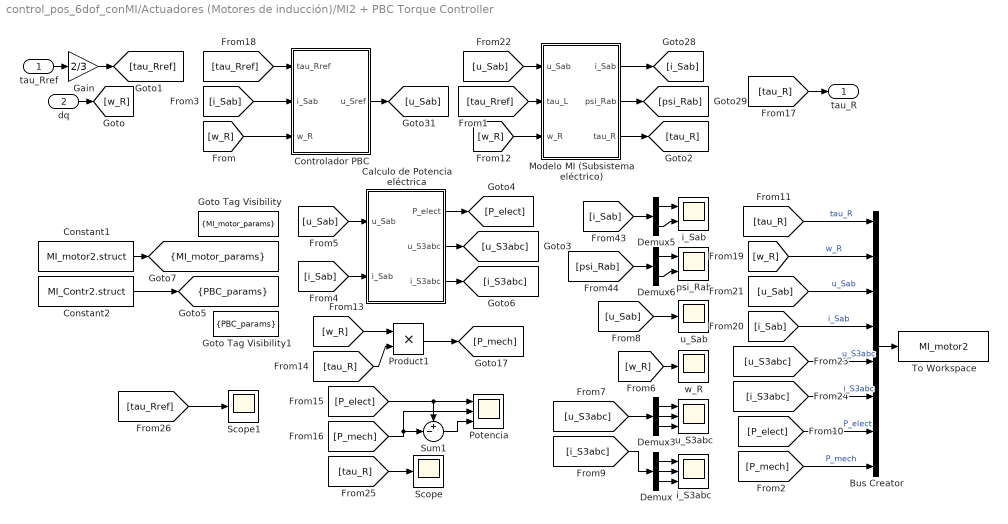
== system control_pos_6dof_conMI/Actuadores (Motores de inducción)/MI2 + PBC Torque Controller ==
  tau_Rref : Inport
  dq : Inport  Port=2
  Bus Creator : BusCreator  Inputs=8
  Calculo de Potencia eléctrica : Subsystem
  Constant1 : Constant  Value=MI_motor2.struct  OutDataTypeStr=Bus: MI_bus
  Constant2 : Constant  Value=MI_Contr2.struct  OutDataTypeStr=Bus: PBC_bus
  Controlador PBC : Subsystem
  Demux : Demux  Outputs=3
  Demux3 : Demux  Outputs=3
  Demux5 : Demux  Outputs=2
  Demux6 : Demux  Outputs=2
  Gain : Gain  Gain=2/3
  Goto Tag Visibility : GotoTagVisibility  GotoTag=MI_motor_params
  Goto Tag Visibility1 : GotoTagVisibility  GotoTag=PBC_params
  Modelo MI (Subsistema eléctrico) : Subsystem
  Potencia : Scope  NumInputPorts=3
  Product1 : Product
  Scope : Scope
  Scope1 : Scope
  Sum1 : Sum  Inputs=+-|
  To Workspace : ToWorkspace  VariableName=MI_motor2  SaveFormat=Timeseries  SampleTime=-1
  i_S3abc : Scope  NumInputPorts=3
  i_Sab : Scope  NumInputPorts=2
  psi_Rab : Scope  NumInputPorts=2
  u_S3abc : Scope  NumInputPorts=3
  u_Sab : Scope
  w_R : Scope
  tau_R : Outport
  tag scope: MI_motor_params=scoped, PBC_params=scoped
  wires:
  Modelo MI (Subsistema eléctrico)/2(psi_Rab) -> [psi_Rab]
  [u_Sab] -> Modelo MI (Subsistema eléctrico)/1(u_Sab)
  [i_Sab] -> Controlador PBC/2(i_Sab)
  Controlador PBC/1(u_Sref) -> [u_Sab]
  [w_R] -> Controlador PBC/3(w_R)
  [tau_Rref] -> Modelo MI (Subsistema eléctrico)/2(tau_L)
  Calculo de Potencia eléctrica/2(u_S3abc) -> [u_S3abc]
  Calculo de Potencia eléctrica/1(P_elect) -> [P_elect]
  Demux5/1 -> i_Sab/1
  [w_R] -> w_R/1
  [u_Sab] -> Calculo de Potencia eléctrica/1(u_Sab)
  [psi_Rab] -> Demux6/1
  [u_Sab] -> u_Sab/1
  Demux6/1 -> psi_Rab/1
  Calculo de Potencia eléctrica/3(i_S3abc) -> [i_S3abc]
  Demux6/2 -> psi_Rab/2
  Demux5/2 -> i_Sab/2
  [i_Sab] -> Calculo de Potencia eléctrica/2(i_Sab)
  [i_Sab] -> Demux5/1
  Demux/2 -> i_S3abc/2
  Demux3/1 -> u_S3abc/1
  Demux3/3 -> u_S3abc/3
  [i_S3abc] -> Demux/1
  Demux/1 -> i_S3abc/1
  Demux/3 -> i_S3abc/3
  [u_S3abc] -> Demux3/1
  Demux3/2 -> u_S3abc/2
  Modelo MI (Subsistema eléctrico)/1(i_Sab) -> [i_Sab]
  Modelo MI (Subsistema eléctrico)/3(tau_R) -> [tau_R]
  Product1/1 -> [P_mech]
  [w_R] -> Product1/1
  [tau_R] -> Product1/2
  [tau_R] -> Bus Creator/1  "tau_R"
  Sum1/1 -> Potencia/3
  [P_elect] -> Potencia/1, Sum1/1
  [P_mech] -> Potencia/2, Sum1/2
  [tau_R] -> tau_R/1
  dq/1 -> [w_R]
  [tau_Rref] -> Controlador PBC/1(tau_Rref)
  [w_R] -> Modelo MI (Subsistema eléctrico)/3(w_R)
  Bus Creator/1 -> To Workspace/1
  Constant1/1 -> [MI_motor_params]
  [tau_R] -> Scope/1
  Constant2/1 -> [PBC_params]
  [w_R] -> Bus Creator/2  "w_R"
  [u_Sab] -> Bus Creator/3  "u_Sab"
  [i_Sab] -> Bus Creator/4  "i_Sab"
  [u_S3abc] -> Bus Creator/5  "u_S3abc"
  [i_S3abc] -> Bus Creator/6  "i_S3abc"
  [P_elect] -> Bus Creator/7  "P_elect"
  [P_mech] -> Bus Creator/8  "P_mech"
  [tau_Rref] -> Scope1/1
  Gain/1 -> [tau_Rref]
  tau_Rref/1 -> Gain/1

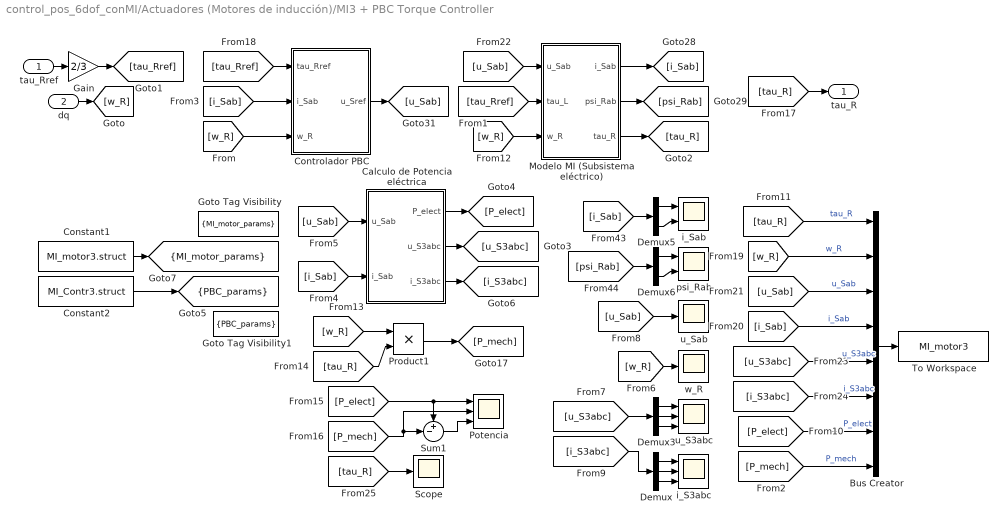
== system control_pos_6dof_conMI/Actuadores (Motores de inducción)/MI3 + PBC Torque Controller ==
  tau_Rref : Inport
  dq : Inport  Port=2
  Bus Creator : BusCreator  Inputs=8
  Calculo de Potencia eléctrica : Subsystem
  Constant1 : Constant  Value=MI_motor3.struct  OutDataTypeStr=Bus: MI_bus
  Constant2 : Constant  Value=MI_Contr3.struct  OutDataTypeStr=Bus: PBC_bus
  Controlador PBC : Subsystem
  Demux : Demux  Outputs=3
  Demux3 : Demux  Outputs=3
  Demux5 : Demux  Outputs=2
  Demux6 : Demux  Outputs=2
  Gain : Gain  Gain=2/3
  Goto Tag Visibility : GotoTagVisibility  GotoTag=MI_motor_params
  Goto Tag Visibility1 : GotoTagVisibility  GotoTag=PBC_params
  Modelo MI (Subsistema eléctrico) : Subsystem
  Potencia : Scope  NumInputPorts=3
  Product1 : Product
  Scope : Scope
  Sum1 : Sum  Inputs=+-|
  To Workspace : ToWorkspace  VariableName=MI_motor3  SaveFormat=Timeseries  SampleTime=-1
  i_S3abc : Scope  NumInputPorts=3
  i_Sab : Scope  NumInputPorts=2
  psi_Rab : Scope  NumInputPorts=2
  u_S3abc : Scope  NumInputPorts=3
  u_Sab : Scope
  w_R : Scope
  tau_R : Outport
  tag scope: MI_motor_params=scoped, PBC_params=scoped
  wires:
  Modelo MI (Subsistema eléctrico)/2(psi_Rab) -> [psi_Rab]
  [u_Sab] -> Modelo MI (Subsistema eléctrico)/1(u_Sab)
  [i_Sab] -> Controlador PBC/2(i_Sab)
  Controlador PBC/1(u_Sref) -> [u_Sab]
  [w_R] -> Controlador PBC/3(w_R)
  [tau_Rref] -> Modelo MI (Subsistema eléctrico)/2(tau_L)
  Calculo de Potencia eléctrica/2(u_S3abc) -> [u_S3abc]
  Calculo de Potencia eléctrica/1(P_elect) -> [P_elect]
  Demux5/1 -> i_Sab/1
  [w_R] -> w_R/1
  [u_Sab] -> Calculo de Potencia eléctrica/1(u_Sab)
  [psi_Rab] -> Demux6/1
  [u_Sab] -> u_Sab/1
  Demux6/1 -> psi_Rab/1
  Calculo de Potencia eléctrica/3(i_S3abc) -> [i_S3abc]
  Demux6/2 -> psi_Rab/2
  Demux5/2 -> i_Sab/2
  [i_Sab] -> Calculo de Potencia eléctrica/2(i_Sab)
  [i_Sab] -> Demux5/1
  Demux/2 -> i_S3abc/2
  Demux3/1 -> u_S3abc/1
  Demux3/3 -> u_S3abc/3
  [i_S3abc] -> Demux/1
  Demux/1 -> i_S3abc/1
  Demux/3 -> i_S3abc/3
  [u_S3abc] -> Demux3/1
  Demux3/2 -> u_S3abc/2
  Modelo MI (Subsistema eléctrico)/1(i_Sab) -> [i_Sab]
  Modelo MI (Subsistema eléctrico)/3(tau_R) -> [tau_R]
  Product1/1 -> [P_mech]
  [w_R] -> Product1/1
  [tau_R] -> Product1/2
  [tau_R] -> Bus Creator/1  "tau_R"
  Sum1/1 -> Potencia/3
  [P_elect] -> Potencia/1, Sum1/1
  [P_mech] -> Potencia/2, Sum1/2
  [tau_R] -> tau_R/1
  dq/1 -> [w_R]
  [tau_Rref] -> Controlador PBC/1(tau_Rref)
  [w_R] -> Modelo MI (Subsistema eléctrico)/3(w_R)
  Bus Creator/1 -> To Workspace/1
  Constant1/1 -> [MI_motor_params]
  [tau_R] -> Scope/1
  Constant2/1 -> [PBC_params]
  [w_R] -> Bus Creator/2  "w_R"
  [u_Sab] -> Bus Creator/3  "u_Sab"
  [i_Sab] -> Bus Creator/4  "i_Sab"
  [u_S3abc] -> Bus Creator/5  "u_S3abc"
  [i_S3abc] -> Bus Creator/6  "i_S3abc"
  [P_elect] -> Bus Creator/7  "P_elect"
  [P_mech] -> Bus Creator/8  "P_mech"
  Gain/1 -> [tau_Rref]
  tau_Rref/1 -> Gain/1

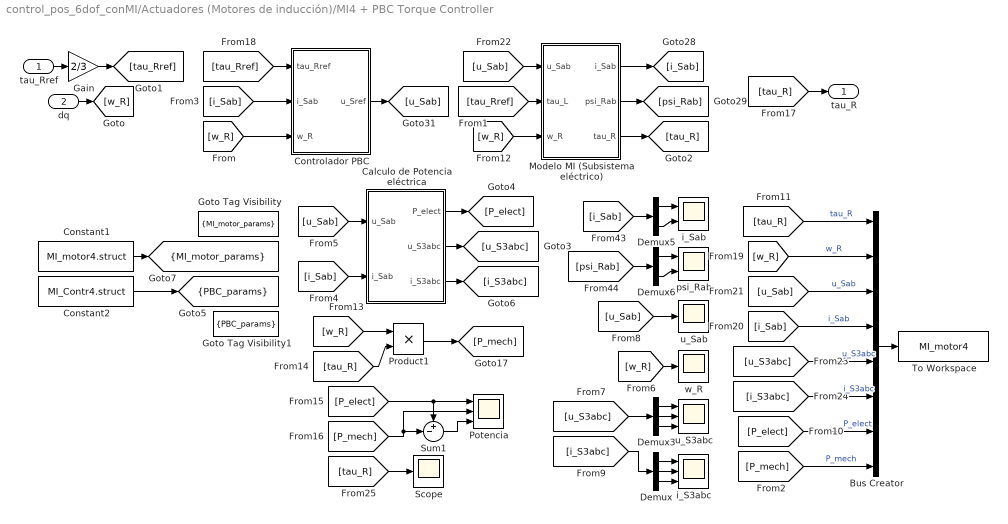
== system control_pos_6dof_conMI/Actuadores (Motores de inducción)/MI4 + PBC Torque Controller ==
  tau_Rref : Inport
  dq : Inport  Port=2
  Bus Creator : BusCreator  Inputs=8
  Calculo de Potencia eléctrica : Subsystem
  Constant1 : Constant  Value=MI_motor4.struct  OutDataTypeStr=Bus: MI_bus
  Constant2 : Constant  Value=MI_Contr4.struct  OutDataTypeStr=Bus: PBC_bus
  Controlador PBC : Subsystem
  Demux : Demux  Outputs=3
  Demux3 : Demux  Outputs=3
  Demux5 : Demux  Outputs=2
  Demux6 : Demux  Outputs=2
  Gain : Gain  Gain=2/3
  Goto Tag Visibility : GotoTagVisibility  GotoTag=MI_motor_params
  Goto Tag Visibility1 : GotoTagVisibility  GotoTag=PBC_params
  Modelo MI (Subsistema eléctrico) : Subsystem
  Potencia : Scope  NumInputPorts=3
  Product1 : Product
  Scope : Scope
  Sum1 : Sum  Inputs=+-|
  To Workspace : ToWorkspace  VariableName=MI_motor4  SaveFormat=Timeseries  SampleTime=-1
  i_S3abc : Scope  NumInputPorts=3
  i_Sab : Scope  NumInputPorts=2
  psi_Rab : Scope  NumInputPorts=2
  u_S3abc : Scope  NumInputPorts=3
  u_Sab : Scope
  w_R : Scope
  tau_R : Outport
  tag scope: MI_motor_params=scoped, PBC_params=scoped
  wires:
  Modelo MI (Subsistema eléctrico)/2(psi_Rab) -> [psi_Rab]
  [u_Sab] -> Modelo MI (Subsistema eléctrico)/1(u_Sab)
  [i_Sab] -> Controlador PBC/2(i_Sab)
  Controlador PBC/1(u_Sref) -> [u_Sab]
  [w_R] -> Controlador PBC/3(w_R)
  [tau_Rref] -> Modelo MI (Subsistema eléctrico)/2(tau_L)
  Calculo de Potencia eléctrica/2(u_S3abc) -> [u_S3abc]
  Calculo de Potencia eléctrica/1(P_elect) -> [P_elect]
  Demux5/1 -> i_Sab/1
  [w_R] -> w_R/1
  [u_Sab] -> Calculo de Potencia eléctrica/1(u_Sab)
  [psi_Rab] -> Demux6/1
  [u_Sab] -> u_Sab/1
  Demux6/1 -> psi_Rab/1
  Calculo de Potencia eléctrica/3(i_S3abc) -> [i_S3abc]
  Demux6/2 -> psi_Rab/2
  Demux5/2 -> i_Sab/2
  [i_Sab] -> Calculo de Potencia eléctrica/2(i_Sab)
  [i_Sab] -> Demux5/1
  Demux/2 -> i_S3abc/2
  Demux3/1 -> u_S3abc/1
  Demux3/3 -> u_S3abc/3
  [i_S3abc] -> Demux/1
  Demux/1 -> i_S3abc/1
  Demux/3 -> i_S3abc/3
  [u_S3abc] -> Demux3/1
  Demux3/2 -> u_S3abc/2
  Modelo MI (Subsistema eléctrico)/1(i_Sab) -> [i_Sab]
  Modelo MI (Subsistema eléctrico)/3(tau_R) -> [tau_R]
  Product1/1 -> [P_mech]
  [w_R] -> Product1/1
  [tau_R] -> Product1/2
  [tau_R] -> Bus Creator/1  "tau_R"
  Sum1/1 -> Potencia/3
  [P_elect] -> Potencia/1, Sum1/1
  [P_mech] -> Potencia/2, Sum1/2
  [tau_R] -> tau_R/1
  dq/1 -> [w_R]
  [tau_Rref] -> Controlador PBC/1(tau_Rref)
  [w_R] -> Modelo MI (Subsistema eléctrico)/3(w_R)
  Bus Creator/1 -> To Workspace/1
  Constant1/1 -> [MI_motor_params]
  [tau_R] -> Scope/1
  Constant2/1 -> [PBC_params]
  [w_R] -> Bus Creator/2  "w_R"
  [u_Sab] -> Bus Creator/3  "u_Sab"
  [i_Sab] -> Bus Creator/4  "i_Sab"
  [u_S3abc] -> Bus Creator/5  "u_S3abc"
  [i_S3abc] -> Bus Creator/6  "i_S3abc"
  [P_elect] -> Bus Creator/7  "P_elect"
  [P_mech] -> Bus Creator/8  "P_mech"
  Gain/1 -> [tau_Rref]
  tau_Rref/1 -> Gain/1
